simulink model "arducopter"  (R2019a)
settings: Solver=FixedStepAuto  StartTime=0.0  StopTime=Tsim  FixedStep=0.01  RelTol=1e-3
values from neighbouring files (symbols this model uses):
  g = 9.81    [arducopter_params.m]
  k_p2 = 1.005572    [arducopter_params.m]
  k_r2 = 1.001888    [arducopter_params.m]
  k_y2 = 1.0    (= 1)    [arducopter_params.m]
  Ts = 0.01    [arducopter_params.m]
  vx_kd = 0.0    (= 0)    [arducopter_params.m]
  vx_ki = 0.0    (= 0)    [arducopter_params.m]
  vx_kp = 0.3    [arducopter_params.m]
  vy_kd = 0.0    (= 0)    [arducopter_params.m]
  vy_ki = 0.0    (= 0)    [arducopter_params.m]
  vy_kp = 0.3    [arducopter_params.m]
  wn_p2 = 10.672720    (= 10.67272)    [arducopter_params.m]
  wn_r2 = 12.485386    [arducopter_params.m]
  wn_y2 = 9.875759    [arducopter_params.m]
  x_initial = 0    [arducopter_params.m]
  x_kd = 0.05    [arducopter_params.m]
  x_ki = 0.0    (= 0)    [arducopter_params.m]
  x_kp = 1.4    [arducopter_params.m]
  y_initial = 0    [arducopter_params.m]
  y_kd = 0.05    [arducopter_params.m]
  y_ki = 0.0    (= 0)    [arducopter_params.m]
  y_kp = 1.4    [arducopter_params.m]
  yaw_initial = 0    [arducopter_params.m]
  zeta_p2 = 1.000000    (= 1)    [arducopter_params.m]
  zeta_r2 = 1.000000    (= 1)    [arducopter_params.m]
  zeta_y2 = 1.000000    (= 1)    [arducopter_params.m]
undefined symbols (not defined in the file or in its folder): Ap, Ar, Ay, Bp, Br, By, Cp, Cr, Cy, Dp, Dr, Dy
settings Model: Creator=antun-desktop  LastModifiedBy=antun-desktop

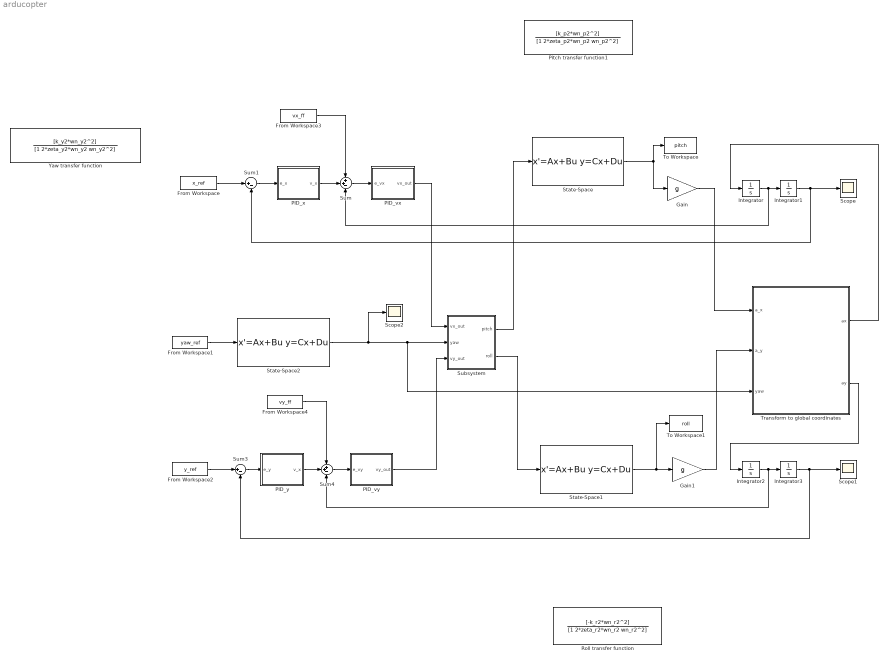
== system arducopter ==
  From Workspace : FromWorkspace  VariableName=x_ref  SampleTime=0
  From Workspace1 : FromWorkspace  VariableName=yaw_ref  SampleTime=0
  From Workspace2 : FromWorkspace  VariableName=y_ref  SampleTime=0
  From Workspace3 : FromWorkspace  VariableName=vx_ff  SampleTime=0
  From Workspace4 : FromWorkspace  VariableName=vy_ff  SampleTime=0
  Gain : Gain  Gain=g
  Gain1 : Gain  Gain=g
  Integrator : Integrator
  Integrator1 : Integrator  InitialCondition=x_initial
  Integrator2 : Integrator
  Integrator3 : Integrator  InitialCondition=y_initial
  PID_vx : Subsystem
  PID_vy : Subsystem
  PID_x : Subsystem
  PID_y : Subsystem
  Pitch transfer function1 : TransferFcn  Numerator=[k_p2*wn_p2^2]  Denominator=[1 2*zeta_p2*wn_p2 wn_p2^2]
  Roll transfer function : TransferFcn  Numerator=[-k_r2*wn_r2^2]  Denominator=[1 2*zeta_r2*wn_r2 wn_r2^2]
  Scope : Scope
  Scope1 : Scope
  Scope2 : Scope
  State-Space : StateSpace  A=Ap  B=Bp  C=Cp  D=Dp  InitialCondition=[0, 0]
  State-Space1 : StateSpace  A=Ar  B=Br  C=Cr  D=Dr  InitialCondition=[0, 0]
  State-Space2 : StateSpace  A=Ay  B=By  C=Cy  D=Dy  InitialCondition=[0; yaw_initial/Cy(2)]
  Subsystem : Subsystem
  Sum : Sum  Inputs=++-
  Sum1 : Sum  Inputs=|+-
  Sum3 : Sum  Inputs=|+-
  Sum4 : Sum  Inputs=++-
  To Workspace : ToWorkspace  VariableName=pitch  SaveFormat=Structure With Time  SampleTime=-1
  To Workspace1 : ToWorkspace  VariableName=roll  SaveFormat=Structure With Time  SampleTime=-1
  Transform to global coordinates : Subsystem
  Yaw transfer function : TransferFcn  Numerator=[k_y2*wn_y2^2]  Denominator=[1 2*zeta_y2*wn_y2 wn_y2^2]
  wires:
  Integrator/1 -> Sum/3, Integrator1/1
  Sum/1 -> PID_vx/1(e_vx)
  Integrator1/1 -> Sum1/2, Scope/1
  From Workspace/1 -> Sum1/1
  Sum1/1 -> PID_x/1(e_x)
  State-Space/1 -> To Workspace/1, Gain/1
  Integrator3/1 -> Scope1/1, Sum3/2
  Sum4/1 -> PID_vy/1(e_vy)
  Sum3/1 -> PID_y/1(e_y)
  State-Space1/1 -> To Workspace1/1, Gain1/1
  Integrator2/1 -> Sum4/3, Integrator3/1
  From Workspace2/1 -> Sum3/1
  PID_y/1(v_x) -> Sum4/2
  From Workspace1/1 -> State-Space2/1
  Gain/1 -> Transform to global coordinates/1(a_x)
  Gain1/1 -> Transform to global coordinates/2(a_y)
  PID_vx/1(vx_out) -> Subsystem/1(vx_out)
  State-Space2/1 -> Scope2/1, Transform to global coordinates/3(yaw), Subsystem/2(yaw)
  PID_vy/1(vy_out) -> Subsystem/3(vy_out)
  Subsystem/2(roll) -> State-Space1/1
  Transform to global coordinates/1(ax) -> Integrator/1
  Transform to global coordinates/2(ay) -> Integrator2/1
  PID_x/1(v_x) -> Sum/2
  From Workspace3/1 -> Sum/1
  From Workspace4/1 -> Sum4/1
  Subsystem/1(pitch) -> State-Space/1

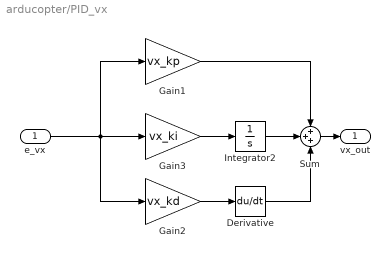
== system arducopter/PID_vx ==
  e_vx : Inport
  Derivative : Derivative
  Gain1 : Gain  Gain=vx_kp
  Gain2 : Gain  Gain=vx_kd
  Gain3 : Gain  Gain=vx_ki
  Integrator2 : Integrator
  Sum : Sum  Inputs=+++
  vx_out : Outport
  wires:
  Gain3/1 -> Integrator2/1
  e_vx/1 -> Gain2/1, Gain1/1, Gain3/1
  Gain1/1 -> Sum/1
  Derivative/1 -> Sum/3
  Integrator2/1 -> Sum/2
  Sum/1 -> vx_out/1
  Gain2/1 -> Derivative/1

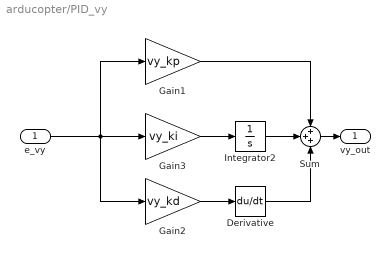
== system arducopter/PID_vy ==
  e_vy : Inport
  Derivative : Derivative
  Gain1 : Gain  Gain=vy_kp
  Gain2 : Gain  Gain=vy_kd
  Gain3 : Gain  Gain=vy_ki
  Integrator2 : Integrator
  Sum : Sum  Inputs=+++
  vy_out : Outport
  wires:
  Gain3/1 -> Integrator2/1
  e_vy/1 -> Gain2/1, Gain1/1, Gain3/1
  Gain1/1 -> Sum/1
  Derivative/1 -> Sum/3
  Integrator2/1 -> Sum/2
  Sum/1 -> vy_out/1
  Gain2/1 -> Derivative/1

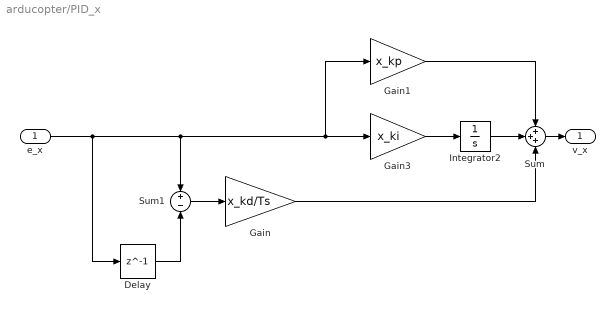
== system arducopter/PID_x ==
  e_x : Inport
  Delay : Delay  DelayLength=1  InitialCondition=0  SampleTime=Ts
  Gain : Gain  Gain=x_kd/Ts
  Gain1 : Gain  Gain=x_kp
  Gain3 : Gain  Gain=x_ki
  Integrator2 : Integrator
  Sum : Sum  Inputs=+++
  Sum1 : Sum  Inputs=+-
  v_x : Outport
  wires:
  Gain3/1 -> Integrator2/1
  e_x/1 -> Delay/1, Gain1/1, Gain3/1, Sum1/1
  Gain1/1 -> Sum/1
  Integrator2/1 -> Sum/2
  Sum/1 -> v_x/1
  Delay/1 -> Sum1/2
  Sum1/1 -> Gain/1
  Gain/1 -> Sum/3

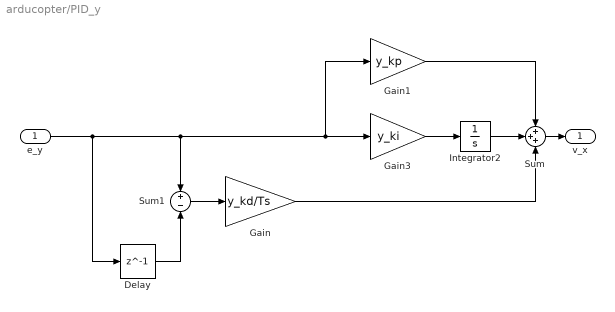
== system arducopter/PID_y ==
  e_y : Inport
  Delay : Delay  DelayLength=1  InitialCondition=0  SampleTime=Ts
  Gain : Gain  Gain=y_kd/Ts
  Gain1 : Gain  Gain=y_kp
  Gain3 : Gain  Gain=y_ki
  Integrator2 : Integrator
  Sum : Sum  Inputs=+++
  Sum1 : Sum  Inputs=+-
  v_x : Outport
  wires:
  Gain3/1 -> Integrator2/1
  e_y/1 -> Delay/1, Gain1/1, Gain3/1, Sum1/1
  Gain1/1 -> Sum/1
  Integrator2/1 -> Sum/2
  Sum/1 -> v_x/1
  Delay/1 -> Sum1/2
  Sum1/1 -> Gain/1
  Gain/1 -> Sum/3

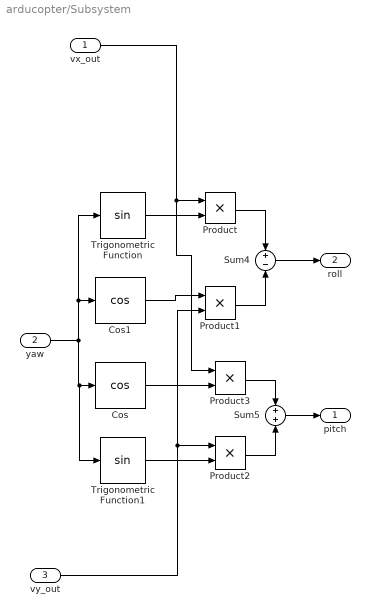
== system arducopter/Subsystem ==
  vx_out : Inport
  yaw : Inport  Port=2
  vy_out : Inport  Port=3
  Cos : Trigonometry  Operator=cos
  Cos1 : Trigonometry  Operator=cos
  Product{,1..3} (4 alike) : Product
  Sum4 : Sum  Inputs=+-
  Sum5 : Sum
  Trigonometric Function : Trigonometry
  Trigonometric Function1 : Trigonometry
  pitch : Outport
  roll : Outport  Port=2
  wires:
  Product2/1 -> Sum5/2
  Product3/1 -> Sum5/1
  yaw/1 -> Trigonometric Function1/1, Cos/1, Trigonometric Function/1, Cos1/1
  Trigonometric Function/1 -> Product/2
  Product/1 -> Sum4/1
  Cos1/1 -> Product1/1
  vy_out/1 -> Product2/1, Product1/2
  Cos/1 -> Product3/2
  Product1/1 -> Sum4/2
  Trigonometric Function1/1 -> Product2/2
  vx_out/1 -> Product3/1, Product/1
  Sum5/1 -> pitch/1
  Sum4/1 -> roll/1

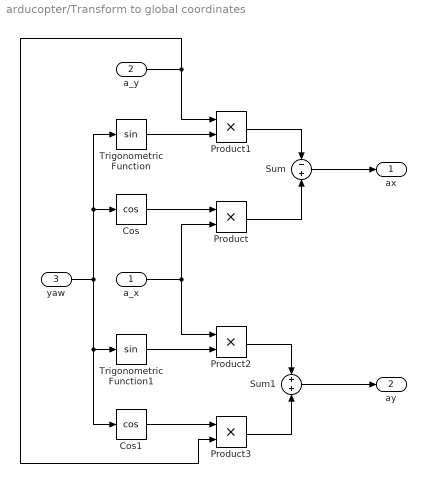
== system arducopter/Transform to global coordinates ==
  a_x : Inport
  a_y : Inport  Port=2
  yaw : Inport  Port=3
  Cos : Trigonometry  Operator=cos
  Cos1 : Trigonometry  Operator=cos
  Product{,1..3} (4 alike) : Product
  Sum : Sum  Inputs=-+
  Sum1 : Sum
  Trigonometric Function : Trigonometry
  Trigonometric Function1 : Trigonometry
  ax : Outport
  ay : Outport  Port=2
  wires:
  Cos/1 -> Product/1
  Trigonometric Function/1 -> Product1/2
  a_x/1 -> Product/2, Product2/1
  Product/1 -> Sum/2
  Product1/1 -> Sum/1
  Sum/1 -> ax/1
  yaw/1 -> Trigonometric Function/1, Cos/1, Cos1/1, Trigonometric Function1/1
  Trigonometric Function1/1 -> Product2/2
  Cos1/1 -> Product3/1
  a_y/1 -> Product3/2, Product1/1
  Product2/1 -> Sum1/1
  Product3/1 -> Sum1/2
  Sum1/1 -> ay/1
